simulink model "car_sim"  (R2020b)
settings: Solver=VariableStepAuto  StartTime=0.01  StopTime=inf  RelTol=1e-3
libraries: etargetslib x2, dspnetwork x2, simulink x1
settings Model: Creator=86150  LastModifiedBy=86150

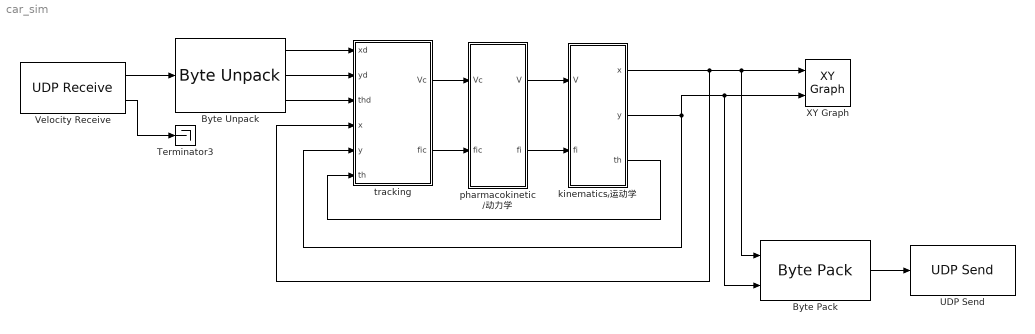
== system car_sim ==
  Byte Pack : etargetslib/Byte Pack  datatypes={'double','double'}  byteAlign=1
  Byte Unpack : etargetslib/Byte Unpack  dimensions={[1],[1],[1]}  datatypes={'double','double','double'}  byteAlign=1
  Terminator3 : Terminator
  UDP Send : dspnetwork/UDP Send  remoteURL='127.0.0.1'  remotePort=25000  localURL='0.0.0.0'  localPortSource=Automatically determine  localPort=-1  sendBufferSize=8192  sampletime=-1  blockPlatform=[]  separateLengthPort=0
  Velocity Receive : dspnetwork/UDP Receive  localURL='0.0.0.0'  localPort=8080  remoteURL='192.168.86.1'  remotePort=-1  recvBufferSize=8192  dims=24  signalDatatype=uint8  isComplex=off  isVarSize=off  showBlockingTime=off  blockingTime=0  sampletime=0.05  blockPlatform=[]
  XY Graph : simulink/Sinks/XY Graph  xmin=-3  xmax=3  ymin=-0.2  ymax=5.2  st=-1
  kinematics/运动学 : Subsystem  mask{L=0.254}
      mask prompts: L "小车车长Ｌ(米)"
  pharmacokinetic /动力学 : Subsystem  mask{Tv=0.1, Tfi=0.1}
      mask prompts: Tv "小车速度驱动时间常数(秒)"; Tfi "小车转向驱动时间常数(秒)"
  tracking : Subsystem
  wires:
  Byte Unpack/3 -> tracking/3(thd)
  Byte Unpack/2 -> tracking/2(yd)
  Byte Unpack/1 -> tracking/1(xd)
  Velocity Receive/2 -> Terminator3/1
  pharmacokinetic /动力学/2(fi) -> kinematics/运动学/2(fi)
  tracking/2(fic) -> pharmacokinetic /动力学/2(fic)
  pharmacokinetic /动力学/1(V) -> kinematics/运动学/1(V)
  Velocity Receive/1 -> Byte Unpack/1
  kinematics/运动学/1(x) -> tracking/4(x), Byte Pack/1, XY Graph/1
  kinematics/运动学/2(y) -> Byte Pack/2, XY Graph/2, tracking/5(y)
  tracking/1(Vc) -> pharmacokinetic /动力学/1(Vc)
  kinematics/运动学/3(th) -> tracking/6(th)
  Byte Pack/1 -> UDP Send/1

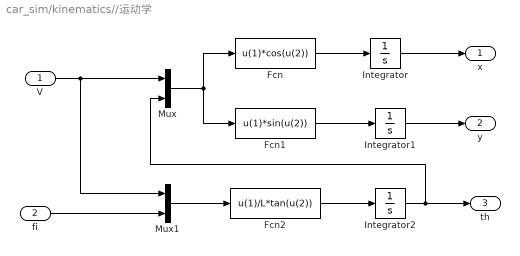
== system car_sim/kinematics//运动学 ==
  V : Inport
  fi : Inport  Port=2
  Fcn : Fcn  Expr=u(1)*cos(u(2))
  Fcn1 : Fcn  Expr=u(1)*sin(u(2))
  Fcn2 : Fcn  Expr=u(1)/L*tan(u(2))
  Integrator : Integrator
  Integrator1 : Integrator
  Integrator2 : Integrator
  Mux : Mux  Inputs=2
  Mux1 : Mux  Inputs=2
  x : Outport
  y : Outport  Port=2
  th : Outport  Port=3
  wires:
  Mux/1 -> Fcn1/1, Fcn/1
  Fcn/1 -> Integrator/1
  Fcn2/1 -> Integrator2/1
  Mux1/1 -> Fcn2/1
  Integrator2/1 -> th/1, Mux/2
  V/1 -> Mux1/1, Mux/1
  Integrator/1 -> x/1
  Integrator1/1 -> y/1
  fi/1 -> Mux1/2
  Fcn1/1 -> Integrator1/1

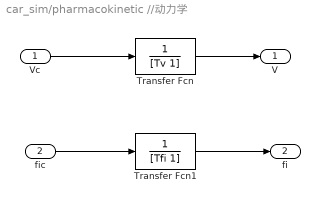
== system car_sim/pharmacokinetic //动力学 ==
  Vc : Inport
  fic : Inport  Port=2
  Transfer Fcn : TransferFcn  Denominator=[Tv 1]
  Transfer Fcn1 : TransferFcn  Denominator=[Tfi 1]
  V : Outport
  fi : Outport  Port=2
  wires:
  Vc/1 -> Transfer Fcn/1
  fic/1 -> Transfer Fcn1/1
  Transfer Fcn1/1 -> fi/1
  Transfer Fcn/1 -> V/1

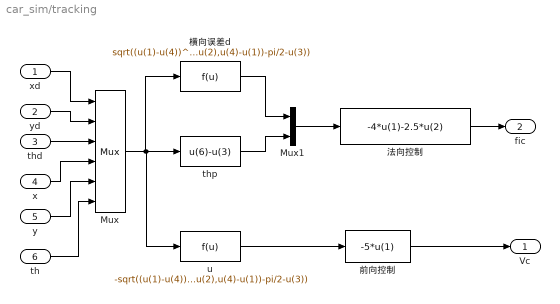
== system car_sim/tracking ==
  xd : Inport
  yd : Inport  Port=2
  thd : Inport  Port=3
  x : Inport  Port=4
  y : Inport  Port=5
  th : Inport  Port=6
  Mux : Mux  Inputs=6
  Mux1 : Mux  Inputs=2
  thp : Fcn  Expr=u(6)-u(3)
  u : Fcn  Expr=-sqrt((u(1)-u(4))^2+(u(2)-u(5))^2)*sin(atan2(u(5)-u(2),u(4)-u(1))-pi/2-u(3))
  前向控制 : Fcn  Expr=-5*u(1)
  横向误差d : Fcn  Expr=sqrt((u(1)-u(4))^2+(u(2)-u(5))^2)*cos(atan2(u(5)-u(2),u(4)-u(1))-pi/2-u(3))
  法向控制 : Fcn  Expr=-4*u(1)-2.5*u(2)
  Vc : Outport
  fic : Outport  Port=2
  wires:
  th/1 -> Mux/6
  xd/1 -> Mux/1
  x/1 -> Mux/4
  thd/1 -> Mux/3
  前向控制/1 -> Vc/1
  y/1 -> Mux/5
  法向控制/1 -> fic/1
  yd/1 -> Mux/2
  Mux/1 -> 横向误差d/1, u/1, thp/1
  横向误差d/1 -> Mux1/1
  Mux1/1 -> 法向控制/1
  thp/1 -> Mux1/2
  u/1 -> 前向控制/1
